simulink model "parte2_eje4_genfiedl"  (R2017b)
settings: Solver=VariableStepAuto  StartTime=0.0  StopTime=30  RelTol=1e-3
values from neighbouring files (symbols this model uses):
  H = 3.5    [parte2_ej2_GeneradorBusInfinito.m]    (also in parte2_ej2_GeneradorBusInfinitoHP.m; parte2_eje2_HPModel.m)
  K1 = 0.7643    [parte2_ej2_GeneradorBusInfinitoHP.m]    (also in parte2_eje2_HPModel.m = Eb*eqo/D*(RT*sin(do)+XTD*cos(do))+Eb*iqo/D*(xq-xpd)*(XTQ*sin)
  K2 = 0.8649    [parte2_ej2_GeneradorBusInfinitoHP.m]    (also in parte2_eje2_HPModel.m = Lads/(Lads+Lfd)*(RT/D*eqo+(XTQ*(xq-xpd)/D+1)*iqo))
  K3 = 0.3230    (= 0.323)    [parte2_ej2_GeneradorBusInfinitoHP.m]    (also in parte2_eje2_HPModel.m = 0.286464655633)
  K4 = 1.4187    [parte2_ej2_GeneradorBusInfinitoHP.m]    (also in parte2_eje2_HPModel.m = Eb/D*(xd-xpd)*(XTQ*sin(do)-RT*cos(do)))
  KD = 10    [parte2_ej2_GeneradorBusInfinito.m]    (also in parte2_ej2_GeneradorBusInfinitoHP.m)
  T3 = 2.365    [parte2_ej2_GeneradorBusInfinitoHP.m]    (also in parte2_eje2_HPModel.m = 2.29171724507)
settings Model: Creator=Admon  LastModifiedBy=Admon

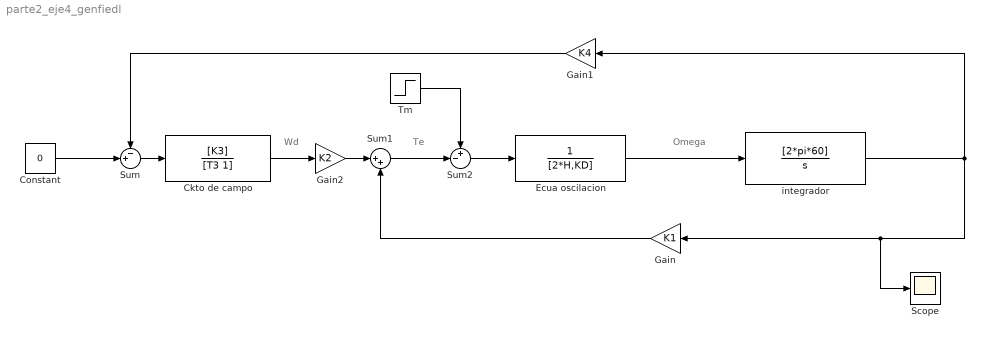
== system parte2_eje4_genfiedl ==
  note: Omega
  note: Te
  note: Wd
  Ckto de campo : TransferFcn  Numerator=[K3]  Denominator=[T3 1]
  Constant : Constant  Value=0
  Ecua oscilacion : TransferFcn  Denominator=[2*H,KD]
  Gain : Gain  Gain=K1
  Gain1 : Gain  Gain=K4
  Gain2 : Gain  Gain=K2
  Scope : Scope
  Sum : Sum  Inputs=-+|
  Sum1 : Sum  Inputs=|++
  Sum2 : Sum  Inputs=+-|
  Tm : Step  SampleTime=0
  integrador : TransferFcn  Numerator=[2*pi*60]  Denominator=[1 0]
  wires:
  Constant/1 -> Sum/2
  Sum/1 -> Ckto de campo/1
  Sum1/1 -> Sum2/2
  Sum2/1 -> Ecua oscilacion/1
  Tm/1 -> Sum2/1
  Ecua oscilacion/1 -> integrador/1
  Ckto de campo/1 -> Gain2/1
  Gain2/1 -> Sum1/1
  integrador/1 -> Scope/1, Gain/1, Gain1/1
  Gain/1 -> Sum1/2
  Gain1/1 -> Sum/1
